simulink model "L2_Step3"  (R2023a)
settings: Solver=FixedStepDiscrete  StartTime=0.0  StopTime=inf  FixedStep=0.01  RelTol=1e-3
model workspace (MATLAB code in the model file):
  | IgnitionOff = 0;
  | IgnitionACC = 1;
  | IgnitionOnEngineOn = 2;
  | 
  | Active = 1;
  | Not_Active = 0;
  | 
  | 
  | Present = 1;
  | Absent = 0;
settings Model: Creator=Ekrem Fidan  LastModifiedBy=okanduzyel
settings DebuggingCC: UnconnectedInputMsg=warning  UnconnectedOutputMsg=warning  UnconnectedLineMsg=warning
settings ModelReferenceCC: EnableRefExpFcnMdlSchedulingChecks=on
settings RTWCC: DLArmComputeVersion=19.05

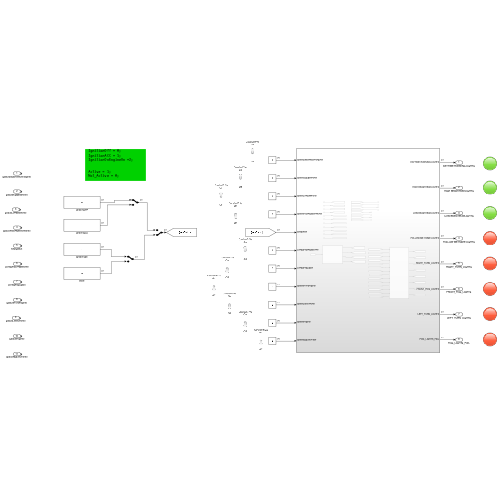
[thumbnail: Simulink's stored preview of the top-level diagram]
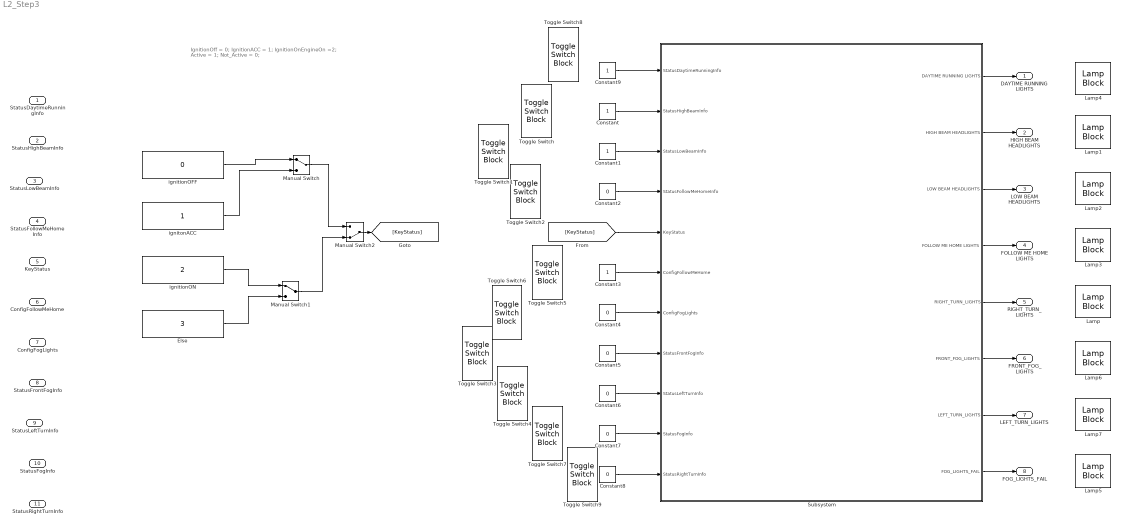
== system L2_Step3 ==
  note: IgnitionOff = 0;
      | IgnitionACC = 1;
      | IgnitionOnEngineOn =2;
      |
      | Active = 1;
      | Not_Active = 0;
  StatusDaytimeRunningInfo : Inport
  StatusHighBeamInfo : Inport  Port=2
  StatusLowBeamInfo : Inport  Port=3
  StatusFollowMeHomeInfo : Inport  Port=4
  KeyStatus : Inport  Port=5
  ConfigFollowMeHome : Inport  Port=6
  ConfigFogLights : Inport  Port=7
  StatusFrontFogInfo : Inport  Port=8
  StatusLeftTurnInfo : Inport  Port=9
  StatusFogInfo : Inport  Port=10
  StatusRightTurnInfo : Inport  Port=11
  Constant{,1,3,9} (4 alike) : Constant
  Constant{2,4..8} (6 alike) : Constant  Value=0
  Else : Constant  Value=3  SampleTime=-1
  Lamp{,1..7} (8 alike) : LampBlock  LabelPosition=Hide
  Manual Switch : ManualSwitch
  Manual Switch1 : ManualSwitch
  Manual Switch2 : ManualSwitch  CurrentSetting=0
  Subsystem : Subsystem
  Toggle Switch{,1..9} (10 alike) : ToggleSwitchBlock
      settings: Values={{'Off', 'On'}, [0 1]}
  ignitionOFF : Constant  Value=0  SampleTime=-1
  ignitionON : Constant  Value=2  SampleTime=-1
  ignitonACC : Constant  SampleTime=-1
  DAYTIME RUNNING LIGHTS : Outport
  HIGH BEAM HEADLIGHTS : Outport  Port=2
  LOW BEAM HEADLIGHTS : Outport  Port=3
  FOLLOW ME HOME LIGHTS : Outport  Port=4
  RIGHT_TURN_LIGHTS : Outport  Port=5
  FRONT_FOG_LIGHTS : Outport  Port=6
  LEFT_TURN_LIGHTS : Outport  Port=7
  FOG_LIGHTS_FAIL : Outport  Port=8
  wires:
  ignitionOFF/1 -> Manual Switch/1
  ignitonACC/1 -> Manual Switch/2
  ignitionON/1 -> Manual Switch1/1
  Else/1 -> Manual Switch1/2
  Manual Switch/1 -> Manual Switch2/1
  Manual Switch1/1 -> Manual Switch2/2
  Manual Switch2/1 -> [KeyStatus]
  Constant9/1 -> Subsystem/1(StatusDaytimeRunningInfo)
  Constant/1 -> Subsystem/2(StatusHighBeamInfo)
  Constant1/1 -> Subsystem/3(StatusLowBeamInfo)
  Constant2/1 -> Subsystem/4(StatusFollowMeHomeInfo)
  [KeyStatus] -> Subsystem/5(KeyStatus)
  Constant3/1 -> Subsystem/6(ConfigFollowMeHome)
  Constant4/1 -> Subsystem/7(ConfigFogLights)
  Constant5/1 -> Subsystem/8(StatusFrontFogInfo)
  Constant6/1 -> Subsystem/9(StatusLeftTurnInfo)
  Constant7/1 -> Subsystem/10(StatusFogInfo)
  Constant8/1 -> Subsystem/11(StatusRightTurnInfo)
  Subsystem/1(DAYTIME RUNNING LIGHTS) -> DAYTIME RUNNING LIGHTS/1
  Subsystem/2(HIGH BEAM HEADLIGHTS) -> HIGH BEAM HEADLIGHTS/1
  Subsystem/3(LOW BEAM HEADLIGHTS) -> LOW BEAM HEADLIGHTS/1
  Subsystem/4(FOLLOW ME HOME LIGHTS) -> FOLLOW ME HOME LIGHTS/1
  Subsystem/5(RIGHT_TURN_LIGHTS) -> RIGHT_TURN_LIGHTS/1
  Subsystem/6(FRONT_FOG_LIGHTS) -> FRONT_FOG_LIGHTS/1
  Subsystem/7(LEFT_TURN_LIGHTS) -> LEFT_TURN_LIGHTS/1
  Subsystem/8(FOG_LIGHTS_FAIL) -> FOG_LIGHTS_FAIL/1

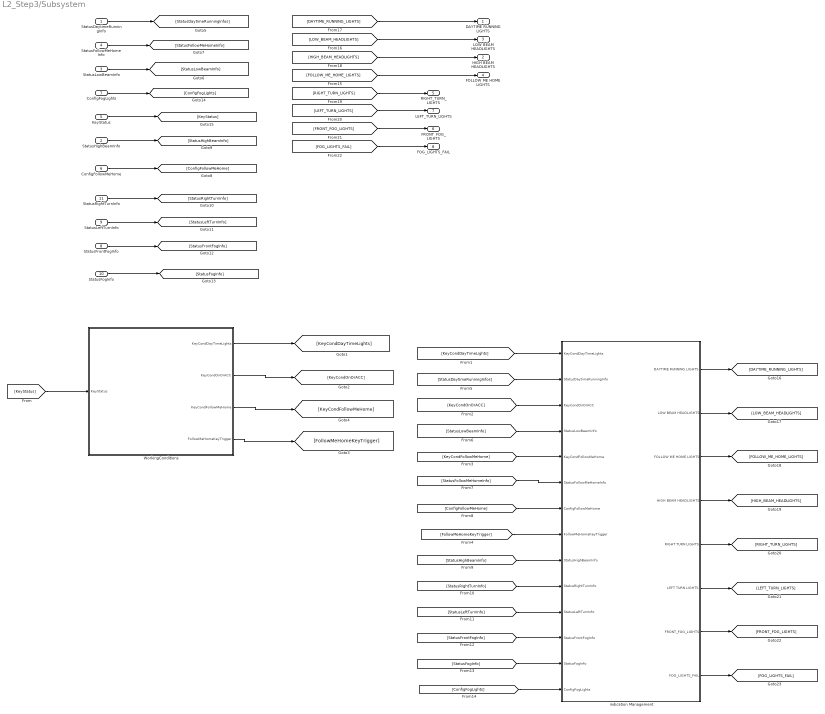
== system L2_Step3/Subsystem ==
  StatusDaytimeRunningInfo : Inport
  StatusHighBeamInfo : Inport  Port=2
  StatusLowBeamInfo : Inport  Port=3
  StatusFollowMeHomeInfo : Inport  Port=4
  KeyStatus : Inport  Port=5
  ConfigFollowMeHome : Inport  Port=6
  ConfigFogLights : Inport  Port=7
  StatusFrontFogInfo : Inport  Port=8
  StatusLeftTurnInfo : Inport  Port=9
  StatusFogInfo : Inport  Port=10
  StatusRightTurnInfo : Inport  Port=11
  WorkingConditions : Subsystem
  indication Management : Subsystem
  DAYTIME RUNNING LIGHTS : Outport
  HIGH BEAM HEADLIGHTS : Outport  Port=2
  LOW BEAM HEADLIGHTS : Outport  Port=3
  FOLLOW ME HOME LIGHTS : Outport  Port=4
  RIGHT_TURN_LIGHTS : Outport  Port=5
  FRONT_FOG_LIGHTS : Outport  Port=6
  LEFT_TURN_LIGHTS : Outport  Port=7
  FOG_LIGHTS_FAIL : Outport  Port=8
  wires:
  WorkingConditions/4(FollowMeHomeKeyTrigger) -> [FollowMeHomeKeyTrigger]
  [ConfigFogLights] -> indication Management/14(ConfigFogLights)
  [StatusFollowMeHomeInfo] -> indication Management/6(StatusFollowMeHomeInfo)
  [FollowMeHomeKeyTrigger] -> indication Management/8(FollowMeHomeKeyTrigger)
  indication Management/8(FOG_LIGHTS_FAIL) -> [FOG_LIGHTS_FAIL]
  [ConfigFollowMeHome] -> indication Management/7(ConfigFollowMeHome)
  [KeyStatus] -> WorkingConditions/1(KeyStatus)
  [KeyCondOnOrACC] -> indication Management/3(KeyCondOnOrACC)
  [StatusLeftTurnInfo] -> indication Management/11(StatusLeftTurnInfo)
  [StatusFrontFogInfo] -> indication Management/12(StatusFrontFogInfo)
  [KeyCondDayTimeLights] -> indication Management/1(KeyCondDayTimeLights)
  indication Management/7(FRONT_FOG_LIGHTS) -> [FRONT_FOG_LIGHTS]
  StatusLowBeamInfo/1 -> [StatusLowBeamInfo]
  [RIGHT_TURN_LIGHTS] -> RIGHT_TURN_LIGHTS/1
  ConfigFollowMeHome/1 -> [ConfigFollowMeHome]
  [StatusLowBeamInfo] -> indication Management/4(StatusLowBeamInfo)
  [KeyCondFollowMeHome] -> indication Management/5(KeyCondFollowMeHome)
  KeyStatus/1 -> [KeyStatus]
  WorkingConditions/3(KeyCondFollowMeHome) -> [KeyCondFollowMeHome]
  StatusDaytimeRunningInfo/1 -> [StatusDaytimeRunningInfos]
  StatusFollowMeHomeInfo/1 -> [StatusFollowMeHomeInfo]
  [StatusFogInfo] -> indication Management/13(StatusFogInfo)
  [LOW_BEAM_HEADLIGHTS] -> LOW BEAM HEADLIGHTS/1
  ConfigFogLights/1 -> [ConfigFogLights]
  StatusFogInfo/1 -> [StatusFogInfo]
  WorkingConditions/2(KeyCondOnOrACC) -> [KeyCondOnOrACC]
  [StatusHighBeamInfo] -> indication Management/9(StatusHighBeamInfo)
  StatusRightTurnInfo/1 -> [StatusRightTurnInfo]
  [HIGH_BEAM_HEADLIGHTS] -> HIGH BEAM HEADLIGHTS/1
  indication Management/5(RIGHT TURN LIGHTS) -> [RIGHT_TURN_LIGHTS]
  StatusHighBeamInfo/1 -> [StatusHighBeamInfo]
  [DAYTIME_RUNNING_LIGHTS] -> DAYTIME RUNNING LIGHTS/1
  indication Management/1(DAYTIME RUNNING LIGHTS) -> [DAYTIME_RUNNING_LIGHTS]
  StatusFrontFogInfo/1 -> [StatusFrontFogInfo]
  indication Management/3(FOLLOW ME HOME LIGHTS) -> [FOLLOW_ME_HOME_LIGHTS]
  [StatusRightTurnInfo] -> indication Management/10(StatusRightTurnInfo)
  [StatusDaytimeRunningInfos] -> indication Management/2(StatusDaytimeRunningInfo)
  indication Management/6(LEFT TURN LIGHTS) -> [LEFT_TURN_LIGHTS]
  WorkingConditions/1(KeyCondDayTimeLights) -> [KeyCondDayTimeLights]
  indication Management/2(LOW BEAM HEADLIGHTS) -> [LOW_BEAM_HEADLIGHTS]
  StatusLeftTurnInfo/1 -> [StatusLeftTurnInfo]
  indication Management/4(HIGH BEAM HEADLIGHTS) -> [HIGH_BEAM_HEADLIGHTS]
  [FRONT_FOG_LIGHTS] -> FRONT_FOG_LIGHTS/1
  [FOLLOW_ME_HOME_LIGHTS] -> FOLLOW ME HOME LIGHTS/1
  [FOG_LIGHTS_FAIL] -> FOG_LIGHTS_FAIL/1
  [LEFT_TURN_LIGHTS] -> LEFT_TURN_LIGHTS/1

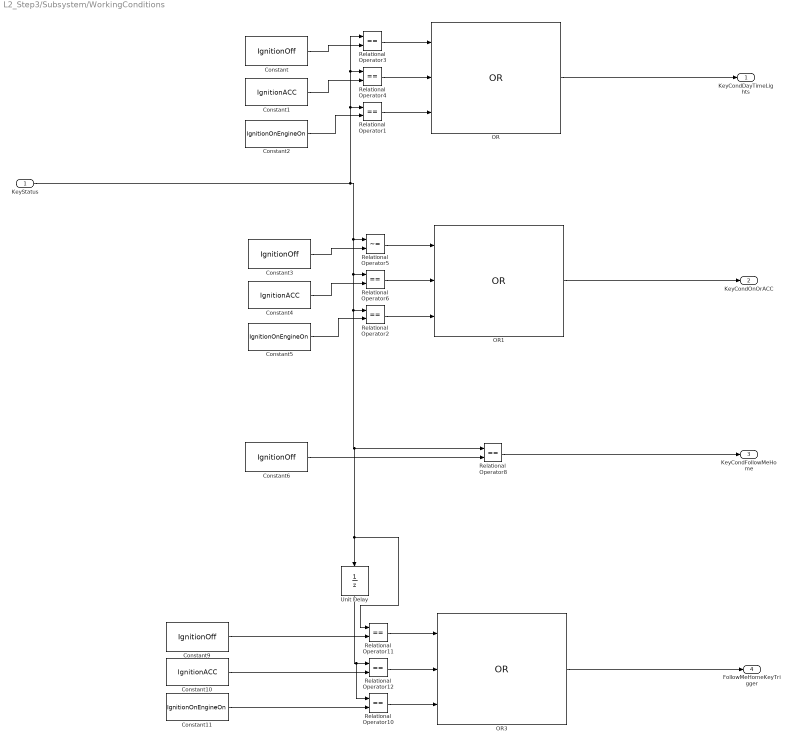
== system L2_Step3/Subsystem/WorkingConditions ==
  KeyStatus : Inport
  Constant{,3,6,9} (4 alike) : Constant  Value=IgnitionOff  SampleTime=-1
  Constant1 : Constant  Value=IgnitionACC  SampleTime=-1
  Constant10 : Constant  Value=IgnitionACC  SampleTime=-1
  Constant11 : Constant  Value=IgnitionOnEngineOn  SampleTime=-1
  Constant2 : Constant  Value=IgnitionOnEngineOn  SampleTime=-1
  Constant4 : Constant  Value=IgnitionACC  SampleTime=-1
  Constant5 : Constant  Value=IgnitionOnEngineOn  SampleTime=-1
  OR : Logic  Operator=OR  Inputs=3  IconShape=distinctive  AllPortsSameDT=off  OutDataTypeStr=boolean
  OR1 : Logic  Operator=OR  Inputs=3  IconShape=distinctive  AllPortsSameDT=off  OutDataTypeStr=boolean
  OR3 : Logic  Operator=OR  Inputs=3  IconShape=distinctive  AllPortsSameDT=off  OutDataTypeStr=boolean
  Relational Operator{1..4,6,8,10..12} (9 alike) : RelationalOperator  Operator===  OutDataTypeStr=boolean  RndMeth=Simplest  InputSameDT=off
  Relational Operator5 : RelationalOperator  Operator=~=  OutDataTypeStr=boolean  RndMeth=Simplest  InputSameDT=off
  Unit Delay : UnitDelay  SampleTime=-1  HasFrameUpgradeWarning=on
  KeyCondDayTimeLights : Outport
  KeyCondOnOrACC : Outport  Port=2
  KeyCondFollowMeHome : Outport  Port=3
  FollowMeHomeKeyTrigger : Outport  Port=4
  wires:
  Constant1/1 -> Relational Operator4/2
  Relational Operator3/1 -> OR/1
  Constant/1 -> Relational Operator3/2
  Relational Operator4/1 -> OR/2
  OR/1 -> KeyCondDayTimeLights/1
  Relational Operator1/1 -> OR/3
  Constant2/1 -> Relational Operator1/2
  Constant5/1 -> Relational Operator2/2
  Relational Operator2/1 -> OR1/3
  OR1/1 -> KeyCondOnOrACC/1
  Relational Operator6/1 -> OR1/2
  Constant3/1 -> Relational Operator5/2
  Relational Operator5/1 -> OR1/1
  Constant4/1 -> Relational Operator6/2
  Constant6/1 -> Relational Operator8/2
  Relational Operator8/1 -> KeyCondFollowMeHome/1
  Constant11/1 -> Relational Operator10/2
  Relational Operator10/1 -> OR3/3
  OR3/1 -> FollowMeHomeKeyTrigger/1
  Relational Operator12/1 -> OR3/2
  Constant9/1 -> Relational Operator11/2
  Relational Operator11/1 -> OR3/1
  KeyStatus/1 -> Relational Operator11/1, Unit Delay/1, Relational Operator8/1, Relational Operator2/1, Relational Operator6/1, Relational Operator5/1, Relational Operator1/1, Relational Operator4/1, Relational Operator3/1
  Constant10/1 -> Relational Operator12/2
  Unit Delay/1 -> Relational Operator10/1, Relational Operator12/1

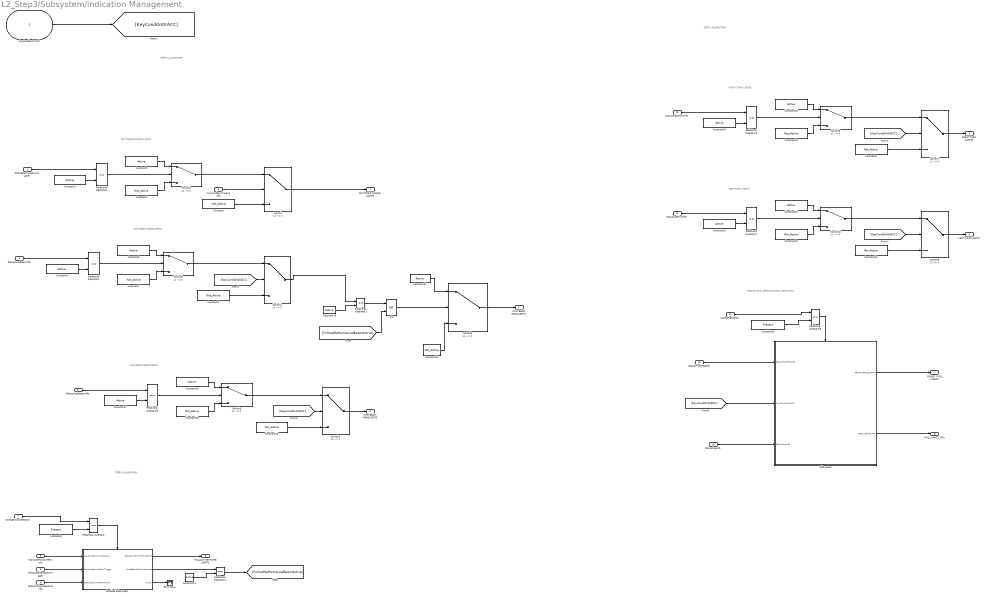
== system L2_Step3/Subsystem/indication Management ==
  note: STEP 1 ALGORITHM
  note: DAYTIME RUNNING LIGHTS
  note: LOW BEAM HEADLIGHTS
  note: HIGH BEAM HEADLIGHTS
  note: RIGHT TURN LIGHTS
  note: LEFT TURN LIGHTS
  note: FRONT FOG LIGHTS and FOG LIGHTS FAIL
  note: STEP 2 ALGORITHM
  note: STEP 3 ALGORITHM
  KeyCondDayTimeLights : Inport
  StatusDaytimeRunningInfo : Inport  Port=2
  KeyCondOnOrACC : Inport  Port=3
  StatusLowBeamInfo : Inport  Port=4
  KeyCondFollowMeHome : Inport  Port=5
  StatusFollowMeHomeInfo : Inport  Port=6
  ConfigFollowMeHome : Inport  Port=7
  FollowMeHomeKeyTrigger : Inport  Port=8
  StatusHighBeamInfo : Inport  Port=9
  StatusRightTurnInfo : Inport  Port=10
  StatusLeftTurnInfo : Inport  Port=11
  StatusFrontFogInfo : Inport  Port=12
  StatusFogInfo : Inport  Port=13
  ConfigFogLights : Inport  Port=14
  Constant{,3..4,7,9,12,16,19..20,23..24} (11 alike) : Constant  Value=Not_Active  SampleTime=-1
  Constant{1..2,5..6,10..11,13..15,17..18,21..22} (13 alike) : Constant  Value=Active  SampleTime=-1
  Constant25 : Constant  Value=Present  SampleTime=-1
  Constant8 : Constant  Value=Present  SampleTime=-1
  Enabled Subsystem : Subsystem  TreatAsAtomicUnit=on
  OR : Logic  Operator=OR  IconShape=distinctive  AllPortsSameDT=off  OutDataTypeStr=boolean
  Relational Operator{,1..8} (9 alike) : RelationalOperator  Operator===  OutDataTypeStr=boolean  RndMeth=Simplest  InputSameDT=off
  Subsystem : Subsystem
  Switch{,1..10} (11 alike) : Switch  Criteria=u2 ~= 0  SaturateOnIntegerOverflow=off  InputSameDT=off
  Terminator : Terminator
  DAYTIME RUNNING LIGHTS : Outport
  LOW BEAM HEADLIGHTS : Outport  Port=2
  FOLLOW ME HOME LIGHTS : Outport  Port=3
  HIGH BEAM HEADLIGHTS : Outport  Port=4
  RIGHT TURN LIGHTS : Outport  Port=5
  LEFT TURN LIGHTS : Outport  Port=6
  FRONT_FOG_LIGHTS : Outport  Port=7
  FOG_LIGHTS_FAIL : Outport  Port=8
  wires:
  Constant1/1 -> Relational Operator3/2
  KeyCondDayTimeLights/1 -> Switch/2
  Switch2/1 -> Switch/1
  Constant2/1 -> Switch2/1
  Switch/1 -> DAYTIME RUNNING LIGHTS/1
  Constant/1 -> Switch/3
  Constant3/1 -> Switch2/3
  Relational Operator3/1 -> Switch2/2
  StatusDaytimeRunningInfo/1 -> Relational Operator3/1
  StatusLowBeamInfo/1 -> Relational Operator1/1
  Relational Operator1/1 -> Switch3/2
  Constant7/1 -> Switch3/3
  Constant4/1 -> Switch1/3
  Switch1/1 -> Relational Operator2/1
  Constant6/1 -> Switch3/1
  Switch3/1 -> Switch1/1
  [KeyCondOnOrACC] -> Switch1/2
  Constant5/1 -> Relational Operator1/2
  Enabled Subsystem/1(FOLLOW ME HOME LIGHTS) -> FOLLOW ME HOME LIGHTS/1
  ConfigFollowMeHome/1 -> Relational Operator/1
  Constant8/1 -> Relational Operator/2
  Relational Operator/1 -> Enabled Subsystem/Enable
  Enabled Subsystem/2(LowBeamFollowMeHome) -> Relational Operator4/1
  Constant14/1 -> Relational Operator4/2
  Constant13/1 -> Relational Operator2/2
  Constant11/1 -> Switch5/1
  Constant12/1 -> Switch5/3
  Relational Operator2/1 -> OR/1
  [FollowMeHomeLowBeamActive] -> OR/2
  OR/1 -> Switch5/2
  Switch5/1 -> LOW BEAM HEADLIGHTS/1
  StatusFollowMeHomeInfo/1 -> Enabled Subsystem/3(StatusFollowMeHomeInfo)
  FollowMeHomeKeyTrigger/1 -> Enabled Subsystem/2(FollowMeHomeKeyTrigger)
  KeyCondFollowMeHome/1 -> Enabled Subsystem/1(KeyCondFollowMeHome)
  Enabled Subsystem/3(timer) -> Terminator/1
  KeyCondOnOrACC/1 -> [KeyCondOnOrACC]
  Relational Operator4/1 -> [FollowMeHomeLowBeamActive]
  Constant17/1 -> Relational Operator5/2
  [KeyCondOnOrACC] -> Switch4/2
  Switch6/1 -> Switch4/1
  Constant18/1 -> Switch6/1
  Constant16/1 -> Switch4/3
  Constant19/1 -> Switch6/3
  Relational Operator5/1 -> Switch6/2
  StatusHighBeamInfo/1 -> Relational Operator5/1
  Switch4/1 -> HIGH BEAM HEADLIGHTS/1
  Switch7/1 -> RIGHT TURN LIGHTS/1
  Constant9/1 -> Switch7/3
  StatusRightTurnInfo/1 -> Relational Operator6/1
  Constant20/1 -> Switch8/3
  Relational Operator6/1 -> Switch8/2
  Constant10/1 -> Relational Operator6/2
  Switch8/1 -> Switch7/1
  Constant15/1 -> Switch8/1
  [KeyCondOnOrACC] -> Switch7/2
  [KeyCondOnOrACC] -> Switch9/2
  Constant22/1 -> Switch10/1
  Switch10/1 -> Switch9/1
  Constant21/1 -> Relational Operator7/2
  Relational Operator7/1 -> Switch10/2
  Constant23/1 -> Switch10/3
  StatusLeftTurnInfo/1 -> Relational Operator7/1
  Constant24/1 -> Switch9/3
  Switch9/1 -> LEFT TURN LIGHTS/1
  StatusFrontFogInfo/1 -> Subsystem/1(StatusFrontFogInfo)
  [KeyCondOnOrACC] -> Subsystem/2(KeyCondOnOrACC)
  StatusFogInfo/1 -> Subsystem/3(StatusFogInfo)
  Subsystem/1(FRONT_FOG_LIGHTS) -> FRONT_FOG_LIGHTS/1
  Subsystem/2(FOG LIGHTS FAIL) -> FOG_LIGHTS_FAIL/1
  ConfigFogLights/1 -> Relational Operator8/1
  Constant25/1 -> Relational Operator8/2
  Relational Operator8/1 -> Subsystem/Enable

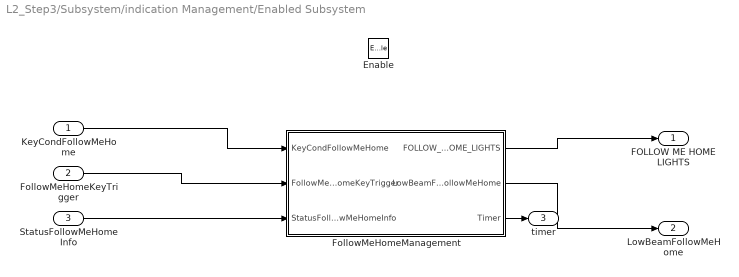
== system L2_Step3/Subsystem/indication Management/Enabled Subsystem ==
  KeyCondFollowMeHome : Inport
  FollowMeHomeKeyTrigger : Inport  Port=2
  StatusFollowMeHomeInfo : Inport  Port=3
  Enable : EnablePort
  FollowMeHomeManagement : Stateflow chart  TreatAsAtomicUnit=on
  FOLLOW ME HOME LIGHTS : Outport  InitialOutput=Not_Active
  LowBeamFollowMeHome : Outport  Port=2  InitialOutput=Not_Active
  timer : Outport  Port=3  InitialOutput=Not_Active
  wires:
  FollowMeHomeKeyTrigger/1 -> FollowMeHomeManagement/2(FollowMeHomeKeyTrigger)
  StatusFollowMeHomeInfo/1 -> FollowMeHomeManagement/3(StatusFollowMeHomeInfo)
  KeyCondFollowMeHome/1 -> FollowMeHomeManagement/1(KeyCondFollowMeHome)
  FollowMeHomeManagement/1(FOLLOW_ME_HOME_LIGHTS) -> FOLLOW ME HOME LIGHTS/1
  FollowMeHomeManagement/2(LowBeamFollowMeHome) -> LowBeamFollowMeHome/1
  FollowMeHomeManagement/3(Timer) -> timer/1

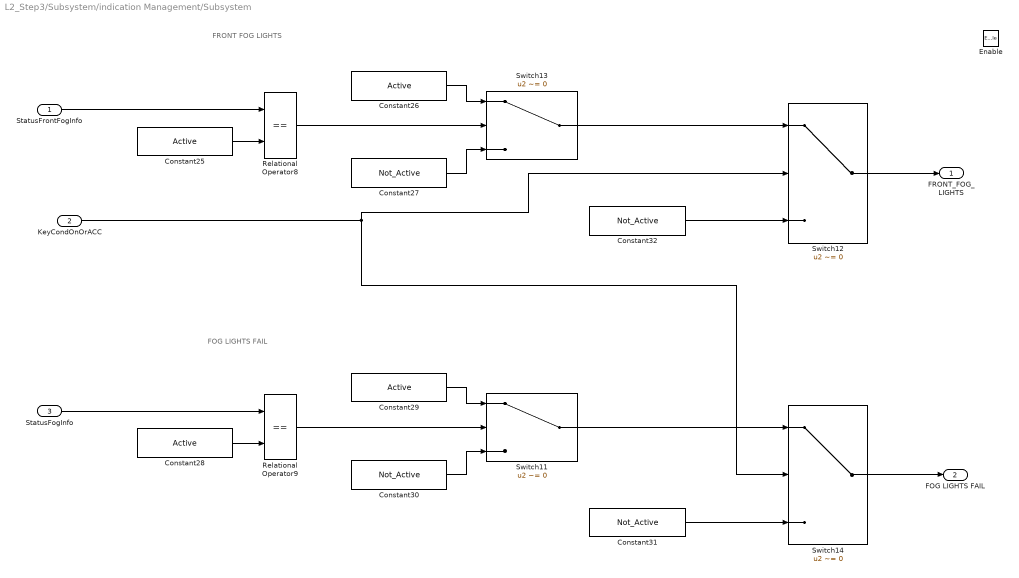
== system L2_Step3/Subsystem/indication Management/Subsystem ==
  note: FOG LIGHTS FAIL
  note: FRONT FOG LIGHTS
  StatusFrontFogInfo : Inport
  KeyCondOnOrACC : Inport  Port=2
  StatusFogInfo : Inport  Port=3
  Enable : EnablePort
  Constant{25..26,28..29} (4 alike) : Constant  Value=Active  SampleTime=-1
  Constant{27,30..32} (4 alike) : Constant  Value=Not_Active  SampleTime=-1
  Relational Operator8 : RelationalOperator  Operator===  OutDataTypeStr=boolean  RndMeth=Simplest  InputSameDT=off
  Relational Operator9 : RelationalOperator  Operator===  OutDataTypeStr=boolean  RndMeth=Simplest  InputSameDT=off
  Switch{11..14} (4 alike) : Switch  Criteria=u2 ~= 0  SaturateOnIntegerOverflow=off  InputSameDT=off
  FRONT_FOG_LIGHTS : Outport
  FOG LIGHTS FAIL : Outport  Port=2
  wires:
  Constant28/1 -> Relational Operator9/2
  Constant25/1 -> Relational Operator8/2
  Constant30/1 -> Switch11/3
  Constant31/1 -> Switch14/3
  StatusFrontFogInfo/1 -> Relational Operator8/1
  Constant32/1 -> Switch12/3
  Switch11/1 -> Switch14/1
  Switch12/1 -> FRONT_FOG_LIGHTS/1
  Constant29/1 -> Switch11/1
  KeyCondOnOrACC/1 -> Switch12/2, Switch14/2
  Constant26/1 -> Switch13/1
  Switch13/1 -> Switch12/1
  Constant27/1 -> Switch13/3
  Relational Operator8/1 -> Switch13/2
  Switch14/1 -> FOG LIGHTS FAIL/1
  Relational Operator9/1 -> Switch11/2
  StatusFogInfo/1 -> Relational Operator9/1

== stateflow chart L2_Step3/Subsystem/indication Management/Enabled Subsystem/FollowMeHomeManagement ==
  state State_NotActive
    en:
    Timer = 0;
    FOLLOW_ME_HOME_LIGHTS = Not_Active;
    LowBeamFollowMeHome = Not_Active;
    du:
  state State_Active
    en:
    Timer++;
    FOLLOW_ME_HOME_LIGHTS = Active;
    LowBeamFollowMeHome = Active;
    du:
    Timer++;
  note: Ts=0.01 sec
      | T = 30 sec
      | N = T/Ts (30/0.01) = 3000
  (default) -> State_NotActive
  State_Active -> State_NotActive : [Timer>=500  || ...
      |  !KeyCondFollowMeHome || ...
      |  StatusFollowMeHomeInfo == Not_Active]
  State_NotActive -> State_Active : [FollowMeHomeKeyTrigger ...
      | && StatusFollowMeHomeInfo == Active]
  data: KeyCondFollowMeHome input; FollowMeHomeKeyTrigger input; StatusFollowMeHomeInfo input; FOLLOW_ME_HOME_LIGHTS output; LowBeamFollowMeHome output; Active parameter; Not_Active parameter; Timer output double
